simulink model "TST_CoEng_StEng"  (R2016b)
settings: Solver=FixedStepDiscrete  StartTime=0.0  StopTime=simTime  FixedStep=sampleTime  RelTol=1e-3
values from neighbouring files (symbols this model uses):
  testCase = 1    [initTST_CoEng_StEng_001.m]    (also in initTST_CoEng_StEng_002.m = 2; initTST_CoEng_StEng_003.m = 3; initTST_CoEng_StEng_004.m = 4; initTST_CoEng_StEng_005.m = 5)
libraries: simulink x41, UnitTest_Lib x25
(part 1 of 2)
settings Model: Creator=zhengjinyan  LastModifiedBy=zhengjinyan
settings DebuggingCC: SignalRangeChecking=error

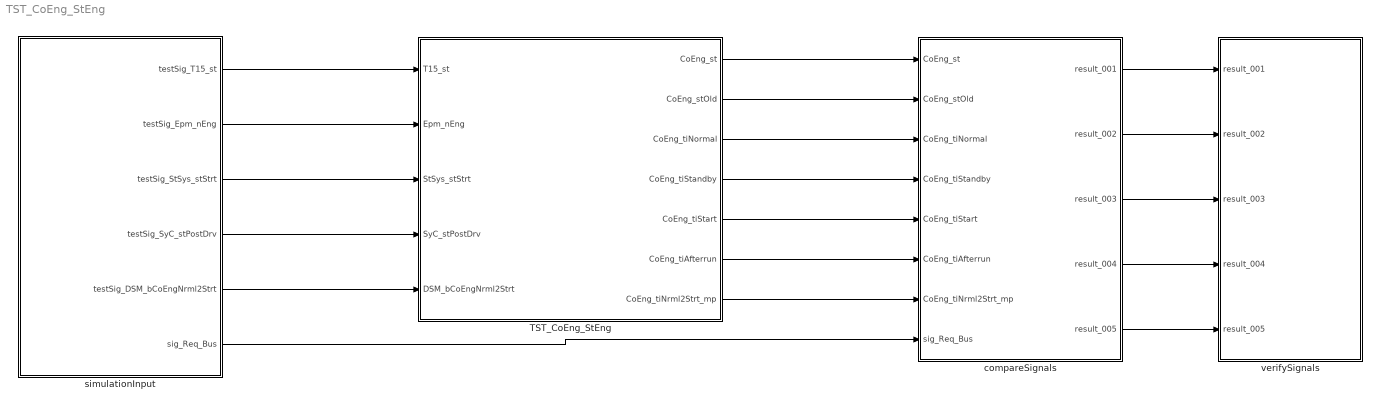
== system TST_CoEng_StEng ==
  TST_CoEng_StEng : Subsystem
  compareSignals : Subsystem
  simulationInput : Subsystem
  verifySignals : Subsystem
  wires:
  simulationInput/1(testSig_T15_st) -> TST_CoEng_StEng/1(T15_st)
  simulationInput/2(testSig_Epm_nEng) -> TST_CoEng_StEng/2(Epm_nEng)
  simulationInput/3(testSig_StSys_stStrt) -> TST_CoEng_StEng/3(StSys_stStrt)
  simulationInput/4(testSig_SyC_stPostDrv) -> TST_CoEng_StEng/4(SyC_stPostDrv)
  simulationInput/5(testSig_DSM_bCoEngNrml2Strt) -> TST_CoEng_StEng/5(DSM_bCoEngNrml2Strt)
  TST_CoEng_StEng/1(CoEng_st) -> compareSignals/1(CoEng_st)
  TST_CoEng_StEng/2(CoEng_stOld) -> compareSignals/2(CoEng_stOld)
  TST_CoEng_StEng/3(CoEng_tiNormal) -> compareSignals/3(CoEng_tiNormal)
  TST_CoEng_StEng/4(CoEng_tiStandby) -> compareSignals/4(CoEng_tiStandby)
  TST_CoEng_StEng/5(CoEng_tiStart) -> compareSignals/5(CoEng_tiStart)
  TST_CoEng_StEng/6(CoEng_tiAfterrun) -> compareSignals/6(CoEng_tiAfterrun)
  TST_CoEng_StEng/7(CoEng_tiNrml2Strt_mp) -> compareSignals/7(CoEng_tiNrml2Strt_mp)
  simulationInput/6(sig_Req_Bus) -> compareSignals/8(sig_Req_Bus)
  compareSignals/1(result_001) -> verifySignals/1(result_001)
  compareSignals/2(result_002) -> verifySignals/2(result_002)
  compareSignals/3(result_003) -> verifySignals/3(result_003)
  compareSignals/4(result_004) -> verifySignals/4(result_004)
  compareSignals/5(result_005) -> verifySignals/5(result_005)

== system TST_CoEng_StEng/TST_CoEng_StEng ==
  T15_st : Inport
  Epm_nEng : Inport  Port=2
  StSys_stStrt : Inport  Port=3
  SyC_stPostDrv : Inport  Port=4
  DSM_bCoEngNrml2Strt : Inport  Port=5
  CoEng_StEng : ModelReference  ModelNameDialog=CoEng_StEng  SimulationMode=Normal  ModelReferenceVersion=1.61  TriggerPortName=function  TriggerPortTriggerType=function-call  TriggerPortStatesWhenEnabling=held
  Function_Call : simulink/Ports & Subsystems/Function-Call Generator  sample_time=sampleTime  numberOfIterations=1
  CoEng_st : Outport
  CoEng_stOld : Outport  Port=2
  CoEng_tiNormal : Outport  Port=3
  CoEng_tiStandby : Outport  Port=4
  CoEng_tiStart : Outport  Port=5
  CoEng_tiAfterrun : Outport  Port=6
  CoEng_tiNrml2Strt_mp : Outport  Port=7
  wires:
  Function_Call/1 -> CoEng_StEng/Trigger
  T15_st/1 -> CoEng_StEng/1
  Epm_nEng/1 -> CoEng_StEng/2
  StSys_stStrt/1 -> CoEng_StEng/3
  SyC_stPostDrv/1 -> CoEng_StEng/4
  DSM_bCoEngNrml2Strt/1 -> CoEng_StEng/5
  CoEng_StEng/1 -> CoEng_st/1
  CoEng_StEng/2 -> CoEng_stOld/1
  CoEng_StEng/3 -> CoEng_tiNormal/1
  CoEng_StEng/4 -> CoEng_tiStandby/1
  CoEng_StEng/5 -> CoEng_tiStart/1
  CoEng_StEng/6 -> CoEng_tiAfterrun/1
  CoEng_StEng/7 -> CoEng_tiNrml2Strt_mp/1

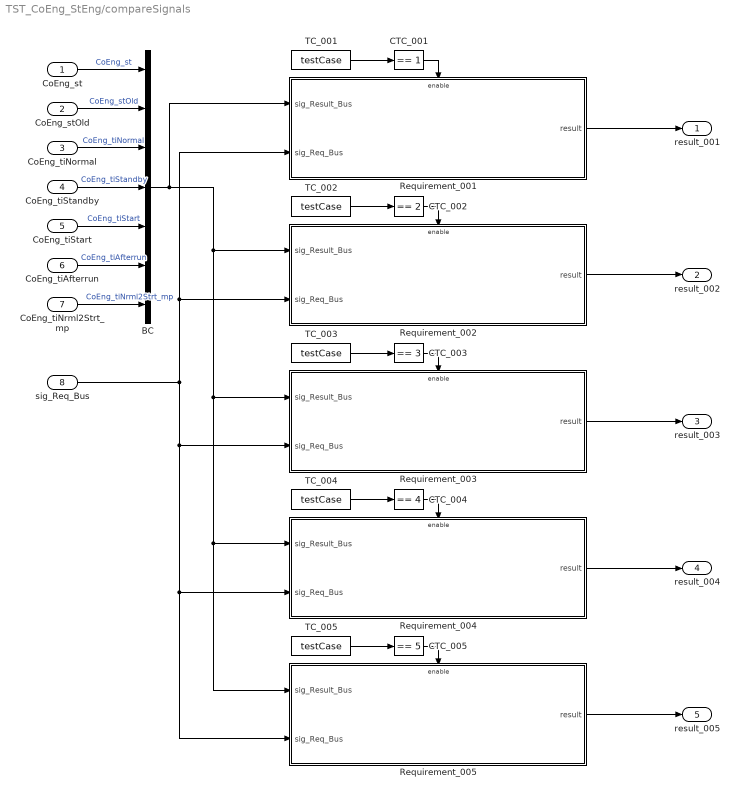
== system TST_CoEng_StEng/compareSignals ==
  CoEng_st : Inport
  CoEng_stOld : Inport  Port=2
  CoEng_tiNormal : Inport  Port=3
  CoEng_tiStandby : Inport  Port=4
  CoEng_tiStart : Inport  Port=5
  CoEng_tiAfterrun : Inport  Port=6
  CoEng_tiNrml2Strt_mp : Inport  Port=7
  sig_Req_Bus : Inport  Port=8
  BC : BusCreator  Inputs=7
  CTC_001 : simulink/Logic and Bit Operations/Compare To Constant  relop===  const=1  OutDataTypeStr=boolean
  CTC_002 : simulink/Logic and Bit Operations/Compare To Constant  relop===  const=2  OutDataTypeStr=boolean
  CTC_003 : simulink/Logic and Bit Operations/Compare To Constant  relop===  const=3  OutDataTypeStr=boolean
  CTC_004 : simulink/Logic and Bit Operations/Compare To Constant  relop===  const=4  OutDataTypeStr=boolean
  CTC_005 : simulink/Logic and Bit Operations/Compare To Constant  relop===  const=5  OutDataTypeStr=boolean
  Requirement_001 : Subsystem
  Requirement_002 : Subsystem
  Requirement_003 : Subsystem
  Requirement_004 : Subsystem
  Requirement_005 : Subsystem
  TC_001 : Constant  Value=testCase
  TC_002 : Constant  Value=testCase
  TC_003 : Constant  Value=testCase
  TC_004 : Constant  Value=testCase
  TC_005 : Constant  Value=testCase
  result_001 : Outport
  result_002 : Outport  Port=2
  result_003 : Outport  Port=3
  result_004 : Outport  Port=4
  result_005 : Outport  Port=5
  wires:
  CoEng_st/1 -> BC/1  "CoEng_st"
  CoEng_stOld/1 -> BC/2  "CoEng_stOld"
  CoEng_tiNormal/1 -> BC/3  "CoEng_tiNormal"
  CoEng_tiStandby/1 -> BC/4  "CoEng_tiStandby"
  CoEng_tiStart/1 -> BC/5  "CoEng_tiStart"
  CoEng_tiAfterrun/1 -> BC/6  "CoEng_tiAfterrun"
  CoEng_tiNrml2Strt_mp/1 -> BC/7  "CoEng_tiNrml2Strt_mp"
  TC_001/1 -> CTC_001/1
  CTC_001/1 -> Requirement_001/Enable
  sig_Req_Bus/1 -> Requirement_004/2(sig_Req_Bus), Requirement_005/2(sig_Req_Bus), Requirement_003/2(sig_Req_Bus), Requirement_001/2(sig_Req_Bus), Requirement_002/2(sig_Req_Bus)
  BC/1 -> Requirement_004/1(sig_Result_Bus), Requirement_005/1(sig_Result_Bus), Requirement_003/1(sig_Result_Bus), Requirement_002/1(sig_Result_Bus), Requirement_001/1(sig_Result_Bus)
  Requirement_001/1(result) -> result_001/1
  TC_002/1 -> CTC_002/1
  CTC_002/1 -> Requirement_002/Enable
  Requirement_002/1(result) -> result_002/1
  TC_003/1 -> CTC_003/1
  CTC_003/1 -> Requirement_003/Enable
  Requirement_003/1(result) -> result_003/1
  TC_004/1 -> CTC_004/1
  CTC_004/1 -> Requirement_004/Enable
  Requirement_004/1(result) -> result_004/1
  TC_005/1 -> CTC_005/1
  CTC_005/1 -> Requirement_005/Enable
  Requirement_005/1(result) -> result_005/1

== system TST_CoEng_StEng/simulationInput ==
  BS : BusSelector  OutputSignals=testSig_T15_st,testSig_Epm_nEng,testSig_StSys_stStrt,testSig_SyC_stPostDrv,testSig_DSM_bCoEngNrml2Strt
  MPSw : MultiPortSwitch  Inputs=5  SaturateOnIntegerOverflow=on  InputSameDT=on
  TestCase : Constant  Value=testCase
  testSignals_R001 : Subsystem
  testSignals_R002 : Subsystem
  testSignals_R003 : Subsystem
  testSignals_R004 : Subsystem
  testSignals_R005 : Subsystem
  testSig_T15_st : Outport
  testSig_Epm_nEng : Outport  Port=2
  testSig_StSys_stStrt : Outport  Port=3
  testSig_SyC_stPostDrv : Outport  Port=4
  testSig_DSM_bCoEngNrml2Strt : Outport  Port=5
  sig_Req_Bus : Outport  Port=6
  wires:
  BS/1 -> testSig_T15_st/1  "<testSig_T15_st>"
  BS/2 -> testSig_Epm_nEng/1  "<testSig_Epm_nEng>"
  BS/3 -> testSig_StSys_stStrt/1  "<testSig_StSys_stStrt>"
  BS/4 -> testSig_SyC_stPostDrv/1  "<testSig_SyC_stPostDrv>"
  BS/5 -> testSig_DSM_bCoEngNrml2Strt/1  "<testSig_DSM_bCoEngNrml2Strt>"
  MPSw/1 -> BS/1, sig_Req_Bus/1
  TestCase/1 -> MPSw/1
  testSignals_R001/1(testSignals) -> MPSw/2
  testSignals_R002/1(testSignals) -> MPSw/3
  testSignals_R003/1(testSignals) -> MPSw/4
  testSignals_R004/1(testSignals) -> MPSw/5
  testSignals_R005/1(testSignals) -> MPSw/6

== system TST_CoEng_StEng/verifySignals ==
  result_001 : Inport
  result_002 : Inport  Port=2
  result_003 : Inport  Port=3
  result_004 : Inport  Port=4
  result_005 : Inport  Port=5
  Assertion_001 : Assertion  Enabled=off
  Assertion_002 : Assertion  Enabled=off
  Assertion_003 : Assertion  Enabled=off
  Assertion_004 : Assertion  Enabled=off
  Assertion_005 : Assertion  Enabled=off
  wires:
  result_001/1 -> Assertion_001/1
  result_002/1 -> Assertion_002/1
  result_003/1 -> Assertion_003/1
  result_004/1 -> Assertion_004/1
  result_005/1 -> Assertion_005/1

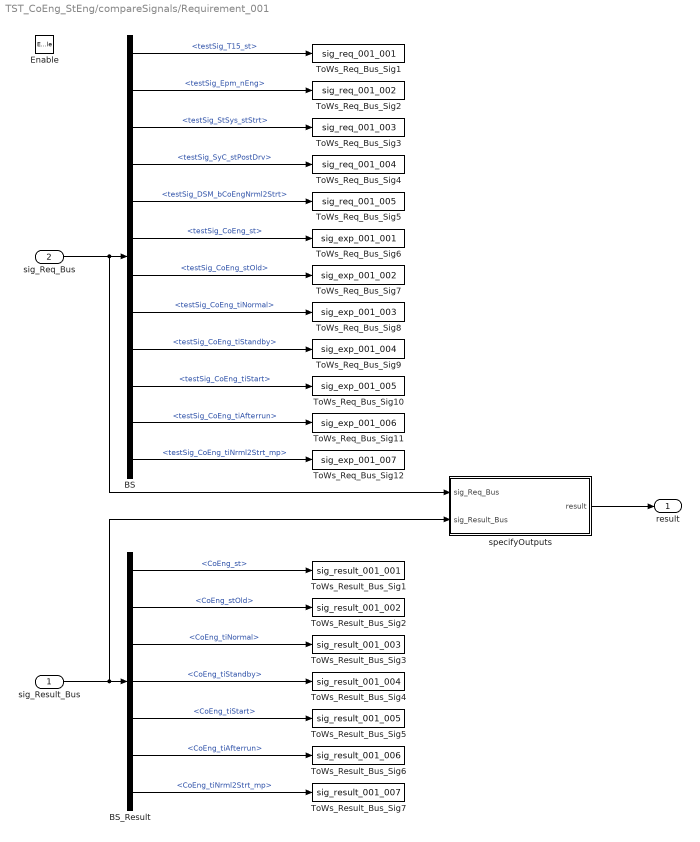
== system TST_CoEng_StEng/compareSignals/Requirement_001 ==
  sig_Result_Bus : Inport
  sig_Req_Bus : Inport  Port=2
  Enable : EnablePort
  BS : BusSelector  OutputSignals=testSig_T15_st,testSig_Epm_nEng,testSig_StSys_stStrt,testSig_SyC_stPostDrv,testSig_DSM_bCoEngNrml2Strt,testSig_CoEng_st,testSig_CoEng_stOld,testSig_CoEng_tiNormal,testSig_CoEng_tiStandby,testSig_CoEng_tiStart,testSig_CoEng_tiAfterrun,testSig_CoEng_tiNrml2Strt_mp
  BS_Result : BusSelector  OutputSignals=CoEng_st,CoEng_stOld,CoEng_tiNormal,CoEng_tiStandby,CoEng_tiStart,CoEng_tiAfterrun,CoEng_tiNrml2Strt_mp
  ToWs_Req_Bus_Sig1 : ToWorkspace  VariableName=sig_req_001_001  SaveFormat=Structure With Time
  ToWs_Req_Bus_Sig10 : ToWorkspace  VariableName=sig_exp_001_005  SaveFormat=Structure With Time
  ToWs_Req_Bus_Sig11 : ToWorkspace  VariableName=sig_exp_001_006  SaveFormat=Structure With Time
  ToWs_Req_Bus_Sig12 : ToWorkspace  VariableName=sig_exp_001_007  SaveFormat=Structure With Time
  ToWs_Req_Bus_Sig2 : ToWorkspace  VariableName=sig_req_001_002  SaveFormat=Structure With Time
  ToWs_Req_Bus_Sig3 : ToWorkspace  VariableName=sig_req_001_003  SaveFormat=Structure With Time
  ToWs_Req_Bus_Sig4 : ToWorkspace  VariableName=sig_req_001_004  SaveFormat=Structure With Time
  ToWs_Req_Bus_Sig5 : ToWorkspace  VariableName=sig_req_001_005  SaveFormat=Structure With Time
  ToWs_Req_Bus_Sig6 : ToWorkspace  VariableName=sig_exp_001_001  SaveFormat=Structure With Time
  ToWs_Req_Bus_Sig7 : ToWorkspace  VariableName=sig_exp_001_002  SaveFormat=Structure With Time
  ToWs_Req_Bus_Sig8 : ToWorkspace  VariableName=sig_exp_001_003  SaveFormat=Structure With Time
  ToWs_Req_Bus_Sig9 : ToWorkspace  VariableName=sig_exp_001_004  SaveFormat=Structure With Time
  ToWs_Result_Bus_Sig1 : ToWorkspace  VariableName=sig_result_001_001  SaveFormat=Structure With Time
  ToWs_Result_Bus_Sig2 : ToWorkspace  VariableName=sig_result_001_002  SaveFormat=Structure With Time
  ToWs_Result_Bus_Sig3 : ToWorkspace  VariableName=sig_result_001_003  SaveFormat=Structure With Time
  ToWs_Result_Bus_Sig4 : ToWorkspace  VariableName=sig_result_001_004  SaveFormat=Structure With Time
  ToWs_Result_Bus_Sig5 : ToWorkspace  VariableName=sig_result_001_005  SaveFormat=Structure With Time
  ToWs_Result_Bus_Sig6 : ToWorkspace  VariableName=sig_result_001_006  SaveFormat=Structure With Time
  ToWs_Result_Bus_Sig7 : ToWorkspace  VariableName=sig_result_001_007  SaveFormat=Structure With Time
  specifyOutputs : Subsystem
  result : Outport
  wires:
  sig_Req_Bus/1 -> BS/1, specifyOutputs/1(sig_Req_Bus)
  BS/1 -> ToWs_Req_Bus_Sig1/1  "<testSig_T15_st>"
  BS/2 -> ToWs_Req_Bus_Sig2/1  "<testSig_Epm_nEng>"
  BS/3 -> ToWs_Req_Bus_Sig3/1  "<testSig_StSys_stStrt>"
  BS/4 -> ToWs_Req_Bus_Sig4/1  "<testSig_SyC_stPostDrv>"
  BS/5 -> ToWs_Req_Bus_Sig5/1  "<testSig_DSM_bCoEngNrml2Strt>"
  BS/6 -> ToWs_Req_Bus_Sig6/1  "<testSig_CoEng_st>"
  BS/7 -> ToWs_Req_Bus_Sig7/1  "<testSig_CoEng_stOld>"
  BS/8 -> ToWs_Req_Bus_Sig8/1  "<testSig_CoEng_tiNormal>"
  BS/9 -> ToWs_Req_Bus_Sig9/1  "<testSig_CoEng_tiStandby>"
  BS/10 -> ToWs_Req_Bus_Sig10/1  "<testSig_CoEng_tiStart>"
  BS/11 -> ToWs_Req_Bus_Sig11/1  "<testSig_CoEng_tiAfterrun>"
  BS/12 -> ToWs_Req_Bus_Sig12/1  "<testSig_CoEng_tiNrml2Strt_mp>"
  sig_Result_Bus/1 -> BS_Result/1, specifyOutputs/2(sig_Result_Bus)
  BS_Result/1 -> ToWs_Result_Bus_Sig1/1  "<CoEng_st>"
  BS_Result/2 -> ToWs_Result_Bus_Sig2/1  "<CoEng_stOld>"
  BS_Result/3 -> ToWs_Result_Bus_Sig3/1  "<CoEng_tiNormal>"
  BS_Result/4 -> ToWs_Result_Bus_Sig4/1  "<CoEng_tiStandby>"
  BS_Result/5 -> ToWs_Result_Bus_Sig5/1  "<CoEng_tiStart>"
  BS_Result/6 -> ToWs_Result_Bus_Sig6/1  "<CoEng_tiAfterrun>"
  BS_Result/7 -> ToWs_Result_Bus_Sig7/1  "<CoEng_tiNrml2Strt_mp>"
  specifyOutputs/1(result) -> result/1

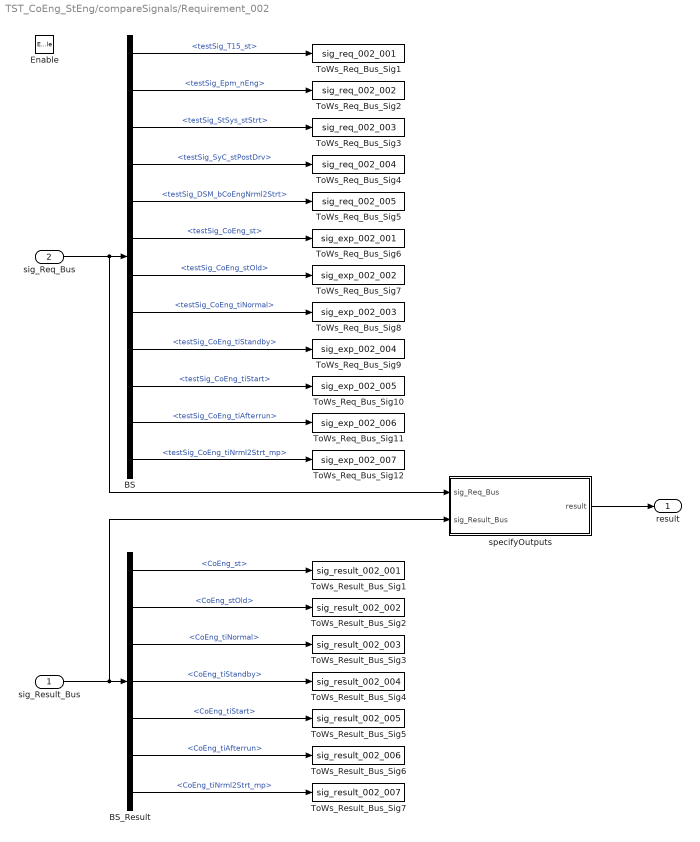
== system TST_CoEng_StEng/compareSignals/Requirement_002 ==
  sig_Result_Bus : Inport
  sig_Req_Bus : Inport  Port=2
  Enable : EnablePort
  BS : BusSelector  OutputSignals=testSig_T15_st,testSig_Epm_nEng,testSig_StSys_stStrt,testSig_SyC_stPostDrv,testSig_DSM_bCoEngNrml2Strt,testSig_CoEng_st,testSig_CoEng_stOld,testSig_CoEng_tiNormal,testSig_CoEng_tiStandby,testSig_CoEng_tiStart,testSig_CoEng_tiAfterrun,testSig_CoEng_tiNrml2Strt_mp
  BS_Result : BusSelector  OutputSignals=CoEng_st,CoEng_stOld,CoEng_tiNormal,CoEng_tiStandby,CoEng_tiStart,CoEng_tiAfterrun,CoEng_tiNrml2Strt_mp
  ToWs_Req_Bus_Sig1 : ToWorkspace  VariableName=sig_req_002_001  SaveFormat=Structure With Time
  ToWs_Req_Bus_Sig10 : ToWorkspace  VariableName=sig_exp_002_005  SaveFormat=Structure With Time
  ToWs_Req_Bus_Sig11 : ToWorkspace  VariableName=sig_exp_002_006  SaveFormat=Structure With Time
  ToWs_Req_Bus_Sig12 : ToWorkspace  VariableName=sig_exp_002_007  SaveFormat=Structure With Time
  ToWs_Req_Bus_Sig2 : ToWorkspace  VariableName=sig_req_002_002  SaveFormat=Structure With Time
  ToWs_Req_Bus_Sig3 : ToWorkspace  VariableName=sig_req_002_003  SaveFormat=Structure With Time
  ToWs_Req_Bus_Sig4 : ToWorkspace  VariableName=sig_req_002_004  SaveFormat=Structure With Time
  ToWs_Req_Bus_Sig5 : ToWorkspace  VariableName=sig_req_002_005  SaveFormat=Structure With Time
  ToWs_Req_Bus_Sig6 : ToWorkspace  VariableName=sig_exp_002_001  SaveFormat=Structure With Time
  ToWs_Req_Bus_Sig7 : ToWorkspace  VariableName=sig_exp_002_002  SaveFormat=Structure With Time
  ToWs_Req_Bus_Sig8 : ToWorkspace  VariableName=sig_exp_002_003  SaveFormat=Structure With Time
  ToWs_Req_Bus_Sig9 : ToWorkspace  VariableName=sig_exp_002_004  SaveFormat=Structure With Time
  ToWs_Result_Bus_Sig1 : ToWorkspace  VariableName=sig_result_002_001  SaveFormat=Structure With Time
  ToWs_Result_Bus_Sig2 : ToWorkspace  VariableName=sig_result_002_002  SaveFormat=Structure With Time
  ToWs_Result_Bus_Sig3 : ToWorkspace  VariableName=sig_result_002_003  SaveFormat=Structure With Time
  ToWs_Result_Bus_Sig4 : ToWorkspace  VariableName=sig_result_002_004  SaveFormat=Structure With Time
  ToWs_Result_Bus_Sig5 : ToWorkspace  VariableName=sig_result_002_005  SaveFormat=Structure With Time
  ToWs_Result_Bus_Sig6 : ToWorkspace  VariableName=sig_result_002_006  SaveFormat=Structure With Time
  ToWs_Result_Bus_Sig7 : ToWorkspace  VariableName=sig_result_002_007  SaveFormat=Structure With Time
  specifyOutputs : Subsystem
  result : Outport
  wires:
  sig_Req_Bus/1 -> BS/1, specifyOutputs/1(sig_Req_Bus)
  BS/1 -> ToWs_Req_Bus_Sig1/1  "<testSig_T15_st>"
  BS/2 -> ToWs_Req_Bus_Sig2/1  "<testSig_Epm_nEng>"
  BS/3 -> ToWs_Req_Bus_Sig3/1  "<testSig_StSys_stStrt>"
  BS/4 -> ToWs_Req_Bus_Sig4/1  "<testSig_SyC_stPostDrv>"
  BS/5 -> ToWs_Req_Bus_Sig5/1  "<testSig_DSM_bCoEngNrml2Strt>"
  BS/6 -> ToWs_Req_Bus_Sig6/1  "<testSig_CoEng_st>"
  BS/7 -> ToWs_Req_Bus_Sig7/1  "<testSig_CoEng_stOld>"
  BS/8 -> ToWs_Req_Bus_Sig8/1  "<testSig_CoEng_tiNormal>"
  BS/9 -> ToWs_Req_Bus_Sig9/1  "<testSig_CoEng_tiStandby>"
  BS/10 -> ToWs_Req_Bus_Sig10/1  "<testSig_CoEng_tiStart>"
  BS/11 -> ToWs_Req_Bus_Sig11/1  "<testSig_CoEng_tiAfterrun>"
  BS/12 -> ToWs_Req_Bus_Sig12/1  "<testSig_CoEng_tiNrml2Strt_mp>"
  sig_Result_Bus/1 -> BS_Result/1, specifyOutputs/2(sig_Result_Bus)
  BS_Result/1 -> ToWs_Result_Bus_Sig1/1  "<CoEng_st>"
  BS_Result/2 -> ToWs_Result_Bus_Sig2/1  "<CoEng_stOld>"
  BS_Result/3 -> ToWs_Result_Bus_Sig3/1  "<CoEng_tiNormal>"
  BS_Result/4 -> ToWs_Result_Bus_Sig4/1  "<CoEng_tiStandby>"
  BS_Result/5 -> ToWs_Result_Bus_Sig5/1  "<CoEng_tiStart>"
  BS_Result/6 -> ToWs_Result_Bus_Sig6/1  "<CoEng_tiAfterrun>"
  BS_Result/7 -> ToWs_Result_Bus_Sig7/1  "<CoEng_tiNrml2Strt_mp>"
  specifyOutputs/1(result) -> result/1

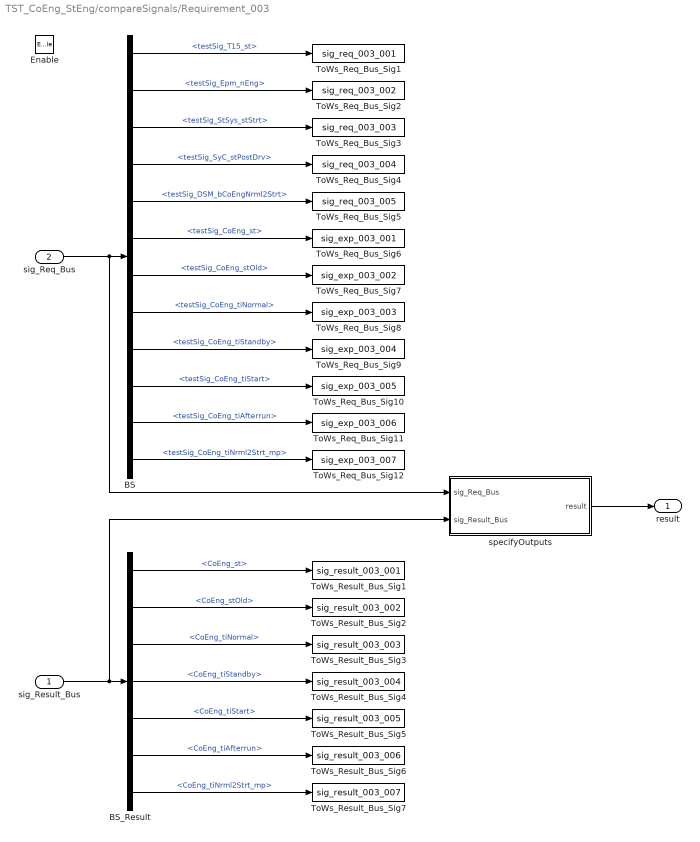
== system TST_CoEng_StEng/compareSignals/Requirement_003 ==
  sig_Result_Bus : Inport
  sig_Req_Bus : Inport  Port=2
  Enable : EnablePort
  BS : BusSelector  OutputSignals=testSig_T15_st,testSig_Epm_nEng,testSig_StSys_stStrt,testSig_SyC_stPostDrv,testSig_DSM_bCoEngNrml2Strt,testSig_CoEng_st,testSig_CoEng_stOld,testSig_CoEng_tiNormal,testSig_CoEng_tiStandby,testSig_CoEng_tiStart,testSig_CoEng_tiAfterrun,testSig_CoEng_tiNrml2Strt_mp
  BS_Result : BusSelector  OutputSignals=CoEng_st,CoEng_stOld,CoEng_tiNormal,CoEng_tiStandby,CoEng_tiStart,CoEng_tiAfterrun,CoEng_tiNrml2Strt_mp
  ToWs_Req_Bus_Sig1 : ToWorkspace  VariableName=sig_req_003_001  SaveFormat=Structure With Time
  ToWs_Req_Bus_Sig10 : ToWorkspace  VariableName=sig_exp_003_005  SaveFormat=Structure With Time
  ToWs_Req_Bus_Sig11 : ToWorkspace  VariableName=sig_exp_003_006  SaveFormat=Structure With Time
  ToWs_Req_Bus_Sig12 : ToWorkspace  VariableName=sig_exp_003_007  SaveFormat=Structure With Time
  ToWs_Req_Bus_Sig2 : ToWorkspace  VariableName=sig_req_003_002  SaveFormat=Structure With Time
  ToWs_Req_Bus_Sig3 : ToWorkspace  VariableName=sig_req_003_003  SaveFormat=Structure With Time
  ToWs_Req_Bus_Sig4 : ToWorkspace  VariableName=sig_req_003_004  SaveFormat=Structure With Time
  ToWs_Req_Bus_Sig5 : ToWorkspace  VariableName=sig_req_003_005  SaveFormat=Structure With Time
  ToWs_Req_Bus_Sig6 : ToWorkspace  VariableName=sig_exp_003_001  SaveFormat=Structure With Time
  ToWs_Req_Bus_Sig7 : ToWorkspace  VariableName=sig_exp_003_002  SaveFormat=Structure With Time
  ToWs_Req_Bus_Sig8 : ToWorkspace  VariableName=sig_exp_003_003  SaveFormat=Structure With Time
  ToWs_Req_Bus_Sig9 : ToWorkspace  VariableName=sig_exp_003_004  SaveFormat=Structure With Time
  ToWs_Result_Bus_Sig1 : ToWorkspace  VariableName=sig_result_003_001  SaveFormat=Structure With Time
  ToWs_Result_Bus_Sig2 : ToWorkspace  VariableName=sig_result_003_002  SaveFormat=Structure With Time
  ToWs_Result_Bus_Sig3 : ToWorkspace  VariableName=sig_result_003_003  SaveFormat=Structure With Time
  ToWs_Result_Bus_Sig4 : ToWorkspace  VariableName=sig_result_003_004  SaveFormat=Structure With Time
  ToWs_Result_Bus_Sig5 : ToWorkspace  VariableName=sig_result_003_005  SaveFormat=Structure With Time
  ToWs_Result_Bus_Sig6 : ToWorkspace  VariableName=sig_result_003_006  SaveFormat=Structure With Time
  ToWs_Result_Bus_Sig7 : ToWorkspace  VariableName=sig_result_003_007  SaveFormat=Structure With Time
  specifyOutputs : Subsystem
  result : Outport
  wires:
  sig_Req_Bus/1 -> BS/1, specifyOutputs/1(sig_Req_Bus)
  BS/1 -> ToWs_Req_Bus_Sig1/1  "<testSig_T15_st>"
  BS/2 -> ToWs_Req_Bus_Sig2/1  "<testSig_Epm_nEng>"
  BS/3 -> ToWs_Req_Bus_Sig3/1  "<testSig_StSys_stStrt>"
  BS/4 -> ToWs_Req_Bus_Sig4/1  "<testSig_SyC_stPostDrv>"
  BS/5 -> ToWs_Req_Bus_Sig5/1  "<testSig_DSM_bCoEngNrml2Strt>"
  BS/6 -> ToWs_Req_Bus_Sig6/1  "<testSig_CoEng_st>"
  BS/7 -> ToWs_Req_Bus_Sig7/1  "<testSig_CoEng_stOld>"
  BS/8 -> ToWs_Req_Bus_Sig8/1  "<testSig_CoEng_tiNormal>"
  BS/9 -> ToWs_Req_Bus_Sig9/1  "<testSig_CoEng_tiStandby>"
  BS/10 -> ToWs_Req_Bus_Sig10/1  "<testSig_CoEng_tiStart>"
  BS/11 -> ToWs_Req_Bus_Sig11/1  "<testSig_CoEng_tiAfterrun>"
  BS/12 -> ToWs_Req_Bus_Sig12/1  "<testSig_CoEng_tiNrml2Strt_mp>"
  sig_Result_Bus/1 -> BS_Result/1, specifyOutputs/2(sig_Result_Bus)
  BS_Result/1 -> ToWs_Result_Bus_Sig1/1  "<CoEng_st>"
  BS_Result/2 -> ToWs_Result_Bus_Sig2/1  "<CoEng_stOld>"
  BS_Result/3 -> ToWs_Result_Bus_Sig3/1  "<CoEng_tiNormal>"
  BS_Result/4 -> ToWs_Result_Bus_Sig4/1  "<CoEng_tiStandby>"
  BS_Result/5 -> ToWs_Result_Bus_Sig5/1  "<CoEng_tiStart>"
  BS_Result/6 -> ToWs_Result_Bus_Sig6/1  "<CoEng_tiAfterrun>"
  BS_Result/7 -> ToWs_Result_Bus_Sig7/1  "<CoEng_tiNrml2Strt_mp>"
  specifyOutputs/1(result) -> result/1

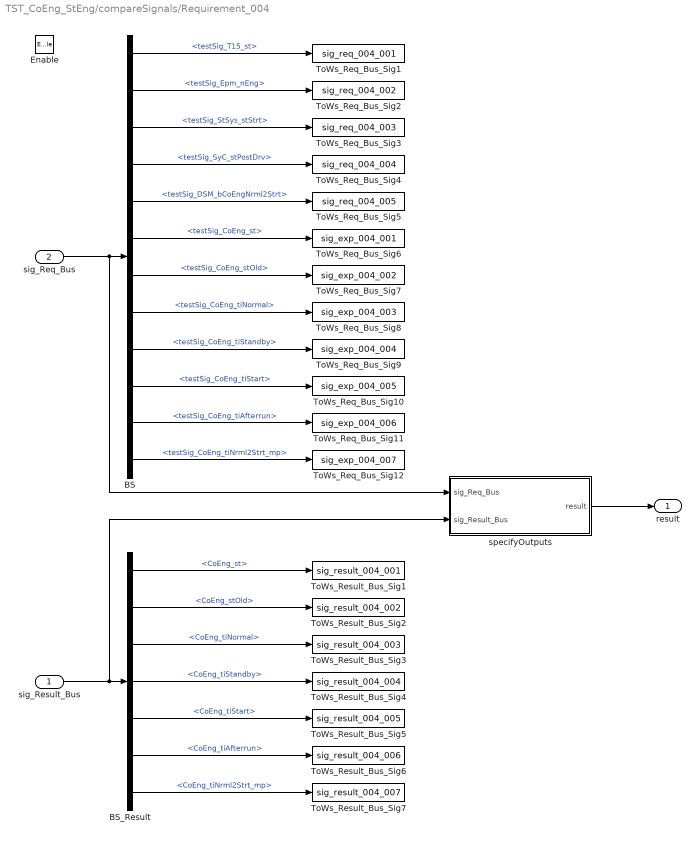
== system TST_CoEng_StEng/compareSignals/Requirement_004 ==
  sig_Result_Bus : Inport
  sig_Req_Bus : Inport  Port=2
  Enable : EnablePort
  BS : BusSelector  OutputSignals=testSig_T15_st,testSig_Epm_nEng,testSig_StSys_stStrt,testSig_SyC_stPostDrv,testSig_DSM_bCoEngNrml2Strt,testSig_CoEng_st,testSig_CoEng_stOld,testSig_CoEng_tiNormal,testSig_CoEng_tiStandby,testSig_CoEng_tiStart,testSig_CoEng_tiAfterrun,testSig_CoEng_tiNrml2Strt_mp
  BS_Result : BusSelector  OutputSignals=CoEng_st,CoEng_stOld,CoEng_tiNormal,CoEng_tiStandby,CoEng_tiStart,CoEng_tiAfterrun,CoEng_tiNrml2Strt_mp
  ToWs_Req_Bus_Sig1 : ToWorkspace  VariableName=sig_req_004_001  SaveFormat=Structure With Time
  ToWs_Req_Bus_Sig10 : ToWorkspace  VariableName=sig_exp_004_005  SaveFormat=Structure With Time
  ToWs_Req_Bus_Sig11 : ToWorkspace  VariableName=sig_exp_004_006  SaveFormat=Structure With Time
  ToWs_Req_Bus_Sig12 : ToWorkspace  VariableName=sig_exp_004_007  SaveFormat=Structure With Time
  ToWs_Req_Bus_Sig2 : ToWorkspace  VariableName=sig_req_004_002  SaveFormat=Structure With Time
  ToWs_Req_Bus_Sig3 : ToWorkspace  VariableName=sig_req_004_003  SaveFormat=Structure With Time
  ToWs_Req_Bus_Sig4 : ToWorkspace  VariableName=sig_req_004_004  SaveFormat=Structure With Time
  ToWs_Req_Bus_Sig5 : ToWorkspace  VariableName=sig_req_004_005  SaveFormat=Structure With Time
  ToWs_Req_Bus_Sig6 : ToWorkspace  VariableName=sig_exp_004_001  SaveFormat=Structure With Time
  ToWs_Req_Bus_Sig7 : ToWorkspace  VariableName=sig_exp_004_002  SaveFormat=Structure With Time
  ToWs_Req_Bus_Sig8 : ToWorkspace  VariableName=sig_exp_004_003  SaveFormat=Structure With Time
  ToWs_Req_Bus_Sig9 : ToWorkspace  VariableName=sig_exp_004_004  SaveFormat=Structure With Time
  ToWs_Result_Bus_Sig1 : ToWorkspace  VariableName=sig_result_004_001  SaveFormat=Structure With Time
  ToWs_Result_Bus_Sig2 : ToWorkspace  VariableName=sig_result_004_002  SaveFormat=Structure With Time
  ToWs_Result_Bus_Sig3 : ToWorkspace  VariableName=sig_result_004_003  SaveFormat=Structure With Time
  ToWs_Result_Bus_Sig4 : ToWorkspace  VariableName=sig_result_004_004  SaveFormat=Structure With Time
  ToWs_Result_Bus_Sig5 : ToWorkspace  VariableName=sig_result_004_005  SaveFormat=Structure With Time
  ToWs_Result_Bus_Sig6 : ToWorkspace  VariableName=sig_result_004_006  SaveFormat=Structure With Time
  ToWs_Result_Bus_Sig7 : ToWorkspace  VariableName=sig_result_004_007  SaveFormat=Structure With Time
  specifyOutputs : Subsystem
  result : Outport
  wires:
  sig_Req_Bus/1 -> BS/1, specifyOutputs/1(sig_Req_Bus)
  BS/1 -> ToWs_Req_Bus_Sig1/1  "<testSig_T15_st>"
  BS/2 -> ToWs_Req_Bus_Sig2/1  "<testSig_Epm_nEng>"
  BS/3 -> ToWs_Req_Bus_Sig3/1  "<testSig_StSys_stStrt>"
  BS/4 -> ToWs_Req_Bus_Sig4/1  "<testSig_SyC_stPostDrv>"
  BS/5 -> ToWs_Req_Bus_Sig5/1  "<testSig_DSM_bCoEngNrml2Strt>"
  BS/6 -> ToWs_Req_Bus_Sig6/1  "<testSig_CoEng_st>"
  BS/7 -> ToWs_Req_Bus_Sig7/1  "<testSig_CoEng_stOld>"
  BS/8 -> ToWs_Req_Bus_Sig8/1  "<testSig_CoEng_tiNormal>"
  BS/9 -> ToWs_Req_Bus_Sig9/1  "<testSig_CoEng_tiStandby>"
  BS/10 -> ToWs_Req_Bus_Sig10/1  "<testSig_CoEng_tiStart>"
  BS/11 -> ToWs_Req_Bus_Sig11/1  "<testSig_CoEng_tiAfterrun>"
  BS/12 -> ToWs_Req_Bus_Sig12/1  "<testSig_CoEng_tiNrml2Strt_mp>"
  sig_Result_Bus/1 -> BS_Result/1, specifyOutputs/2(sig_Result_Bus)
  BS_Result/1 -> ToWs_Result_Bus_Sig1/1  "<CoEng_st>"
  BS_Result/2 -> ToWs_Result_Bus_Sig2/1  "<CoEng_stOld>"
  BS_Result/3 -> ToWs_Result_Bus_Sig3/1  "<CoEng_tiNormal>"
  BS_Result/4 -> ToWs_Result_Bus_Sig4/1  "<CoEng_tiStandby>"
  BS_Result/5 -> ToWs_Result_Bus_Sig5/1  "<CoEng_tiStart>"
  BS_Result/6 -> ToWs_Result_Bus_Sig6/1  "<CoEng_tiAfterrun>"
  BS_Result/7 -> ToWs_Result_Bus_Sig7/1  "<CoEng_tiNrml2Strt_mp>"
  specifyOutputs/1(result) -> result/1

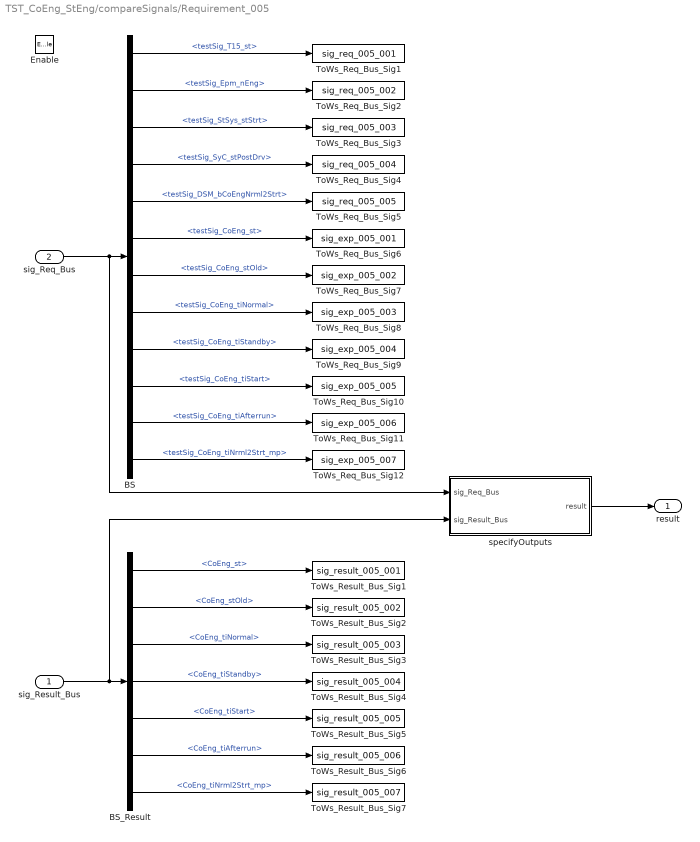
== system TST_CoEng_StEng/compareSignals/Requirement_005 ==
  sig_Result_Bus : Inport
  sig_Req_Bus : Inport  Port=2
  Enable : EnablePort
  BS : BusSelector  OutputSignals=testSig_T15_st,testSig_Epm_nEng,testSig_StSys_stStrt,testSig_SyC_stPostDrv,testSig_DSM_bCoEngNrml2Strt,testSig_CoEng_st,testSig_CoEng_stOld,testSig_CoEng_tiNormal,testSig_CoEng_tiStandby,testSig_CoEng_tiStart,testSig_CoEng_tiAfterrun,testSig_CoEng_tiNrml2Strt_mp
  BS_Result : BusSelector  OutputSignals=CoEng_st,CoEng_stOld,CoEng_tiNormal,CoEng_tiStandby,CoEng_tiStart,CoEng_tiAfterrun,CoEng_tiNrml2Strt_mp
  ToWs_Req_Bus_Sig1 : ToWorkspace  VariableName=sig_req_005_001  SaveFormat=Structure With Time
  ToWs_Req_Bus_Sig10 : ToWorkspace  VariableName=sig_exp_005_005  SaveFormat=Structure With Time
  ToWs_Req_Bus_Sig11 : ToWorkspace  VariableName=sig_exp_005_006  SaveFormat=Structure With Time
  ToWs_Req_Bus_Sig12 : ToWorkspace  VariableName=sig_exp_005_007  SaveFormat=Structure With Time
  ToWs_Req_Bus_Sig2 : ToWorkspace  VariableName=sig_req_005_002  SaveFormat=Structure With Time
  ToWs_Req_Bus_Sig3 : ToWorkspace  VariableName=sig_req_005_003  SaveFormat=Structure With Time
  ToWs_Req_Bus_Sig4 : ToWorkspace  VariableName=sig_req_005_004  SaveFormat=Structure With Time
  ToWs_Req_Bus_Sig5 : ToWorkspace  VariableName=sig_req_005_005  SaveFormat=Structure With Time
  ToWs_Req_Bus_Sig6 : ToWorkspace  VariableName=sig_exp_005_001  SaveFormat=Structure With Time
  ToWs_Req_Bus_Sig7 : ToWorkspace  VariableName=sig_exp_005_002  SaveFormat=Structure With Time
  ToWs_Req_Bus_Sig8 : ToWorkspace  VariableName=sig_exp_005_003  SaveFormat=Structure With Time
  ToWs_Req_Bus_Sig9 : ToWorkspace  VariableName=sig_exp_005_004  SaveFormat=Structure With Time
  ToWs_Result_Bus_Sig1 : ToWorkspace  VariableName=sig_result_005_001  SaveFormat=Structure With Time
  ToWs_Result_Bus_Sig2 : ToWorkspace  VariableName=sig_result_005_002  SaveFormat=Structure With Time
  ToWs_Result_Bus_Sig3 : ToWorkspace  VariableName=sig_result_005_003  SaveFormat=Structure With Time
  ToWs_Result_Bus_Sig4 : ToWorkspace  VariableName=sig_result_005_004  SaveFormat=Structure With Time
  ToWs_Result_Bus_Sig5 : ToWorkspace  VariableName=sig_result_005_005  SaveFormat=Structure With Time
  ToWs_Result_Bus_Sig6 : ToWorkspace  VariableName=sig_result_005_006  SaveFormat=Structure With Time
  ToWs_Result_Bus_Sig7 : ToWorkspace  VariableName=sig_result_005_007  SaveFormat=Structure With Time
  specifyOutputs : Subsystem
  result : Outport
  wires:
  sig_Req_Bus/1 -> BS/1, specifyOutputs/1(sig_Req_Bus)
  BS/1 -> ToWs_Req_Bus_Sig1/1  "<testSig_T15_st>"
  BS/2 -> ToWs_Req_Bus_Sig2/1  "<testSig_Epm_nEng>"
  BS/3 -> ToWs_Req_Bus_Sig3/1  "<testSig_StSys_stStrt>"
  BS/4 -> ToWs_Req_Bus_Sig4/1  "<testSig_SyC_stPostDrv>"
  BS/5 -> ToWs_Req_Bus_Sig5/1  "<testSig_DSM_bCoEngNrml2Strt>"
  BS/6 -> ToWs_Req_Bus_Sig6/1  "<testSig_CoEng_st>"
  BS/7 -> ToWs_Req_Bus_Sig7/1  "<testSig_CoEng_stOld>"
  BS/8 -> ToWs_Req_Bus_Sig8/1  "<testSig_CoEng_tiNormal>"
  BS/9 -> ToWs_Req_Bus_Sig9/1  "<testSig_CoEng_tiStandby>"
  BS/10 -> ToWs_Req_Bus_Sig10/1  "<testSig_CoEng_tiStart>"
  BS/11 -> ToWs_Req_Bus_Sig11/1  "<testSig_CoEng_tiAfterrun>"
  BS/12 -> ToWs_Req_Bus_Sig12/1  "<testSig_CoEng_tiNrml2Strt_mp>"
  sig_Result_Bus/1 -> BS_Result/1, specifyOutputs/2(sig_Result_Bus)
  BS_Result/1 -> ToWs_Result_Bus_Sig1/1  "<CoEng_st>"
  BS_Result/2 -> ToWs_Result_Bus_Sig2/1  "<CoEng_stOld>"
  BS_Result/3 -> ToWs_Result_Bus_Sig3/1  "<CoEng_tiNormal>"
  BS_Result/4 -> ToWs_Result_Bus_Sig4/1  "<CoEng_tiStandby>"
  BS_Result/5 -> ToWs_Result_Bus_Sig5/1  "<CoEng_tiStart>"
  BS_Result/6 -> ToWs_Result_Bus_Sig6/1  "<CoEng_tiAfterrun>"
  BS_Result/7 -> ToWs_Result_Bus_Sig7/1  "<CoEng_tiNrml2Strt_mp>"
  specifyOutputs/1(result) -> result/1

== system TST_CoEng_StEng/simulationInput/testSignals_R001 ==
  BC : BusCreator  Inputs=12
  spec_CoEng_st : FromWorkspace  VariableName=testSig_CoEng_st  Interpolate=off  OutputAfterFinalValue=Holding final value
  spec_CoEng_stOld : FromWorkspace  VariableName=testSig_CoEng_stOld  Interpolate=off  OutputAfterFinalValue=Holding final value
  spec_CoEng_tiAfterrun : FromWorkspace  VariableName=testSig_CoEng_tiAfterrun  Interpolate=off  OutputAfterFinalValue=Holding final value
  spec_CoEng_tiNormal : FromWorkspace  VariableName=testSig_CoEng_tiNormal  Interpolate=off  OutputAfterFinalValue=Holding final value
  spec_CoEng_tiNrml2Strt_mp : FromWorkspace  VariableName=testSig_CoEng_tiNrml2Strt_mp  Interpolate=off  OutputAfterFinalValue=Holding final value
  spec_CoEng_tiStandby : FromWorkspace  VariableName=testSig_CoEng_tiStandby  Interpolate=off  OutputAfterFinalValue=Holding final value
  spec_CoEng_tiStart : FromWorkspace  VariableName=testSig_CoEng_tiStart  Interpolate=off  OutputAfterFinalValue=Holding final value
  spec_DSM_bCoEngNrml2Strt : FromWorkspace  VariableName=testSig_DSM_bCoEngNrml2Strt  Interpolate=off  OutputAfterFinalValue=Holding final value
  spec_Epm_nEng : FromWorkspace  VariableName=testSig_Epm_nEng  Interpolate=off  OutputAfterFinalValue=Holding final value
  spec_StSys_stStrt : FromWorkspace  VariableName=testSig_StSys_stStrt  Interpolate=off  OutputAfterFinalValue=Holding final value
  spec_SyC_stPostDrv : FromWorkspace  VariableName=testSig_SyC_stPostDrv  Interpolate=off  OutputAfterFinalValue=Holding final value
  spec_T15_st : FromWorkspace  VariableName=testSig_T15_st  Interpolate=off  OutputAfterFinalValue=Holding final value
  testSignals : Outport
  wires:
  BC/1 -> testSignals/1
  spec_T15_st/1 -> BC/1  "testSig_T15_st"
  spec_Epm_nEng/1 -> BC/2  "testSig_Epm_nEng"
  spec_StSys_stStrt/1 -> BC/3  "testSig_StSys_stStrt"
  spec_SyC_stPostDrv/1 -> BC/4  "testSig_SyC_stPostDrv"
  spec_DSM_bCoEngNrml2Strt/1 -> BC/5  "testSig_DSM_bCoEngNrml2Strt"
  spec_CoEng_st/1 -> BC/6  "testSig_CoEng_st"
  spec_CoEng_stOld/1 -> BC/7  "testSig_CoEng_stOld"
  spec_CoEng_tiNormal/1 -> BC/8  "testSig_CoEng_tiNormal"
  spec_CoEng_tiStandby/1 -> BC/9  "testSig_CoEng_tiStandby"
  spec_CoEng_tiStart/1 -> BC/10  "testSig_CoEng_tiStart"
  spec_CoEng_tiAfterrun/1 -> BC/11  "testSig_CoEng_tiAfterrun"
  spec_CoEng_tiNrml2Strt_mp/1 -> BC/12  "testSig_CoEng_tiNrml2Strt_mp"

== system TST_CoEng_StEng/simulationInput/testSignals_R002 ==
  BC : BusCreator  Inputs=12
  spec_CoEng_st : FromWorkspace  VariableName=testSig_CoEng_st  Interpolate=off  OutputAfterFinalValue=Holding final value
  spec_CoEng_stOld : FromWorkspace  VariableName=testSig_CoEng_stOld  Interpolate=off  OutputAfterFinalValue=Holding final value
  spec_CoEng_tiAfterrun : FromWorkspace  VariableName=testSig_CoEng_tiAfterrun  Interpolate=off  OutputAfterFinalValue=Holding final value
  spec_CoEng_tiNormal : FromWorkspace  VariableName=testSig_CoEng_tiNormal  Interpolate=off  OutputAfterFinalValue=Holding final value
  spec_CoEng_tiNrml2Strt_mp : FromWorkspace  VariableName=testSig_CoEng_tiNrml2Strt_mp  Interpolate=off  OutputAfterFinalValue=Holding final value
  spec_CoEng_tiStandby : FromWorkspace  VariableName=testSig_CoEng_tiStandby  Interpolate=off  OutputAfterFinalValue=Holding final value
  spec_CoEng_tiStart : FromWorkspace  VariableName=testSig_CoEng_tiStart  Interpolate=off  OutputAfterFinalValue=Holding final value
  spec_DSM_bCoEngNrml2Strt : FromWorkspace  VariableName=testSig_DSM_bCoEngNrml2Strt  Interpolate=off  OutputAfterFinalValue=Holding final value
  spec_Epm_nEng : FromWorkspace  VariableName=testSig_Epm_nEng  Interpolate=off  OutputAfterFinalValue=Holding final value
  spec_StSys_stStrt : FromWorkspace  VariableName=testSig_StSys_stStrt  Interpolate=off  OutputAfterFinalValue=Holding final value
  spec_SyC_stPostDrv : FromWorkspace  VariableName=testSig_SyC_stPostDrv  Interpolate=off  OutputAfterFinalValue=Holding final value
  spec_T15_st : FromWorkspace  VariableName=testSig_T15_st  Interpolate=off  OutputAfterFinalValue=Holding final value
  testSignals : Outport
  wires:
  BC/1 -> testSignals/1
  spec_T15_st/1 -> BC/1  "testSig_T15_st"
  spec_Epm_nEng/1 -> BC/2  "testSig_Epm_nEng"
  spec_StSys_stStrt/1 -> BC/3  "testSig_StSys_stStrt"
  spec_SyC_stPostDrv/1 -> BC/4  "testSig_SyC_stPostDrv"
  spec_DSM_bCoEngNrml2Strt/1 -> BC/5  "testSig_DSM_bCoEngNrml2Strt"
  spec_CoEng_st/1 -> BC/6  "testSig_CoEng_st"
  spec_CoEng_stOld/1 -> BC/7  "testSig_CoEng_stOld"
  spec_CoEng_tiNormal/1 -> BC/8  "testSig_CoEng_tiNormal"
  spec_CoEng_tiStandby/1 -> BC/9  "testSig_CoEng_tiStandby"
  spec_CoEng_tiStart/1 -> BC/10  "testSig_CoEng_tiStart"
  spec_CoEng_tiAfterrun/1 -> BC/11  "testSig_CoEng_tiAfterrun"
  spec_CoEng_tiNrml2Strt_mp/1 -> BC/12  "testSig_CoEng_tiNrml2Strt_mp"

== system TST_CoEng_StEng/simulationInput/testSignals_R003 ==
  BC : BusCreator  Inputs=12
  spec_CoEng_st : FromWorkspace  VariableName=testSig_CoEng_st  Interpolate=off  OutputAfterFinalValue=Holding final value
  spec_CoEng_stOld : FromWorkspace  VariableName=testSig_CoEng_stOld  Interpolate=off  OutputAfterFinalValue=Holding final value
  spec_CoEng_tiAfterrun : FromWorkspace  VariableName=testSig_CoEng_tiAfterrun  Interpolate=off  OutputAfterFinalValue=Holding final value
  spec_CoEng_tiNormal : FromWorkspace  VariableName=testSig_CoEng_tiNormal  Interpolate=off  OutputAfterFinalValue=Holding final value
  spec_CoEng_tiNrml2Strt_mp : FromWorkspace  VariableName=testSig_CoEng_tiNrml2Strt_mp  Interpolate=off  OutputAfterFinalValue=Holding final value
  spec_CoEng_tiStandby : FromWorkspace  VariableName=testSig_CoEng_tiStandby  Interpolate=off  OutputAfterFinalValue=Holding final value
  spec_CoEng_tiStart : FromWorkspace  VariableName=testSig_CoEng_tiStart  Interpolate=off  OutputAfterFinalValue=Holding final value
  spec_DSM_bCoEngNrml2Strt : FromWorkspace  VariableName=testSig_DSM_bCoEngNrml2Strt  Interpolate=off  OutputAfterFinalValue=Holding final value
  spec_Epm_nEng : FromWorkspace  VariableName=testSig_Epm_nEng  Interpolate=off  OutputAfterFinalValue=Holding final value
  spec_StSys_stStrt : FromWorkspace  VariableName=testSig_StSys_stStrt  Interpolate=off  OutputAfterFinalValue=Holding final value
  spec_SyC_stPostDrv : FromWorkspace  VariableName=testSig_SyC_stPostDrv  Interpolate=off  OutputAfterFinalValue=Holding final value
  spec_T15_st : FromWorkspace  VariableName=testSig_T15_st  Interpolate=off  OutputAfterFinalValue=Holding final value
  testSignals : Outport
  wires:
  BC/1 -> testSignals/1
  spec_T15_st/1 -> BC/1  "testSig_T15_st"
  spec_Epm_nEng/1 -> BC/2  "testSig_Epm_nEng"
  spec_StSys_stStrt/1 -> BC/3  "testSig_StSys_stStrt"
  spec_SyC_stPostDrv/1 -> BC/4  "testSig_SyC_stPostDrv"
  spec_DSM_bCoEngNrml2Strt/1 -> BC/5  "testSig_DSM_bCoEngNrml2Strt"
  spec_CoEng_st/1 -> BC/6  "testSig_CoEng_st"
  spec_CoEng_stOld/1 -> BC/7  "testSig_CoEng_stOld"
  spec_CoEng_tiNormal/1 -> BC/8  "testSig_CoEng_tiNormal"
  spec_CoEng_tiStandby/1 -> BC/9  "testSig_CoEng_tiStandby"
  spec_CoEng_tiStart/1 -> BC/10  "testSig_CoEng_tiStart"
  spec_CoEng_tiAfterrun/1 -> BC/11  "testSig_CoEng_tiAfterrun"
  spec_CoEng_tiNrml2Strt_mp/1 -> BC/12  "testSig_CoEng_tiNrml2Strt_mp"

== system TST_CoEng_StEng/simulationInput/testSignals_R004 ==
  BC : BusCreator  Inputs=12
  spec_CoEng_st : FromWorkspace  VariableName=testSig_CoEng_st  Interpolate=off  OutputAfterFinalValue=Holding final value
  spec_CoEng_stOld : FromWorkspace  VariableName=testSig_CoEng_stOld  Interpolate=off  OutputAfterFinalValue=Holding final value
  spec_CoEng_tiAfterrun : FromWorkspace  VariableName=testSig_CoEng_tiAfterrun  Interpolate=off  OutputAfterFinalValue=Holding final value
  spec_CoEng_tiNormal : FromWorkspace  VariableName=testSig_CoEng_tiNormal  Interpolate=off  OutputAfterFinalValue=Holding final value
  spec_CoEng_tiNrml2Strt_mp : FromWorkspace  VariableName=testSig_CoEng_tiNrml2Strt_mp  Interpolate=off  OutputAfterFinalValue=Holding final value
  spec_CoEng_tiStandby : FromWorkspace  VariableName=testSig_CoEng_tiStandby  Interpolate=off  OutputAfterFinalValue=Holding final value
  spec_CoEng_tiStart : FromWorkspace  VariableName=testSig_CoEng_tiStart  Interpolate=off  OutputAfterFinalValue=Holding final value
  spec_DSM_bCoEngNrml2Strt : FromWorkspace  VariableName=testSig_DSM_bCoEngNrml2Strt  Interpolate=off  OutputAfterFinalValue=Holding final value
  spec_Epm_nEng : FromWorkspace  VariableName=testSig_Epm_nEng  Interpolate=off  OutputAfterFinalValue=Holding final value
  spec_StSys_stStrt : FromWorkspace  VariableName=testSig_StSys_stStrt  Interpolate=off  OutputAfterFinalValue=Holding final value
  spec_SyC_stPostDrv : FromWorkspace  VariableName=testSig_SyC_stPostDrv  Interpolate=off  OutputAfterFinalValue=Holding final value
  spec_T15_st : FromWorkspace  VariableName=testSig_T15_st  Interpolate=off  OutputAfterFinalValue=Holding final value
  testSignals : Outport
  wires:
  BC/1 -> testSignals/1
  spec_T15_st/1 -> BC/1  "testSig_T15_st"
  spec_Epm_nEng/1 -> BC/2  "testSig_Epm_nEng"
  spec_StSys_stStrt/1 -> BC/3  "testSig_StSys_stStrt"
  spec_SyC_stPostDrv/1 -> BC/4  "testSig_SyC_stPostDrv"
  spec_DSM_bCoEngNrml2Strt/1 -> BC/5  "testSig_DSM_bCoEngNrml2Strt"
  spec_CoEng_st/1 -> BC/6  "testSig_CoEng_st"
  spec_CoEng_stOld/1 -> BC/7  "testSig_CoEng_stOld"
  spec_CoEng_tiNormal/1 -> BC/8  "testSig_CoEng_tiNormal"
  spec_CoEng_tiStandby/1 -> BC/9  "testSig_CoEng_tiStandby"
  spec_CoEng_tiStart/1 -> BC/10  "testSig_CoEng_tiStart"
  spec_CoEng_tiAfterrun/1 -> BC/11  "testSig_CoEng_tiAfterrun"
  spec_CoEng_tiNrml2Strt_mp/1 -> BC/12  "testSig_CoEng_tiNrml2Strt_mp"

== system TST_CoEng_StEng/simulationInput/testSignals_R005 ==
  BC : BusCreator  Inputs=12
  spec_CoEng_st : FromWorkspace  VariableName=testSig_CoEng_st  Interpolate=off  OutputAfterFinalValue=Holding final value
  spec_CoEng_stOld : FromWorkspace  VariableName=testSig_CoEng_stOld  Interpolate=off  OutputAfterFinalValue=Holding final value
  spec_CoEng_tiAfterrun : FromWorkspace  VariableName=testSig_CoEng_tiAfterrun  Interpolate=off  OutputAfterFinalValue=Holding final value
  spec_CoEng_tiNormal : FromWorkspace  VariableName=testSig_CoEng_tiNormal  Interpolate=off  OutputAfterFinalValue=Holding final value
  spec_CoEng_tiNrml2Strt_mp : FromWorkspace  VariableName=testSig_CoEng_tiNrml2Strt_mp  Interpolate=off  OutputAfterFinalValue=Holding final value
  spec_CoEng_tiStandby : FromWorkspace  VariableName=testSig_CoEng_tiStandby  Interpolate=off  OutputAfterFinalValue=Holding final value
  spec_CoEng_tiStart : FromWorkspace  VariableName=testSig_CoEng_tiStart  Interpolate=off  OutputAfterFinalValue=Holding final value
  spec_DSM_bCoEngNrml2Strt : FromWorkspace  VariableName=testSig_DSM_bCoEngNrml2Strt  Interpolate=off  OutputAfterFinalValue=Holding final value
  spec_Epm_nEng : FromWorkspace  VariableName=testSig_Epm_nEng  Interpolate=off  OutputAfterFinalValue=Holding final value
  spec_StSys_stStrt : FromWorkspace  VariableName=testSig_StSys_stStrt  Interpolate=off  OutputAfterFinalValue=Holding final value
  spec_SyC_stPostDrv : FromWorkspace  VariableName=testSig_SyC_stPostDrv  Interpolate=off  OutputAfterFinalValue=Holding final value
  spec_T15_st : FromWorkspace  VariableName=testSig_T15_st  Interpolate=off  OutputAfterFinalValue=Holding final value
  testSignals : Outport
  wires:
  BC/1 -> testSignals/1
  spec_T15_st/1 -> BC/1  "testSig_T15_st"
  spec_Epm_nEng/1 -> BC/2  "testSig_Epm_nEng"
  spec_StSys_stStrt/1 -> BC/3  "testSig_StSys_stStrt"
  spec_SyC_stPostDrv/1 -> BC/4  "testSig_SyC_stPostDrv"
  spec_DSM_bCoEngNrml2Strt/1 -> BC/5  "testSig_DSM_bCoEngNrml2Strt"
  spec_CoEng_st/1 -> BC/6  "testSig_CoEng_st"
  spec_CoEng_stOld/1 -> BC/7  "testSig_CoEng_stOld"
  spec_CoEng_tiNormal/1 -> BC/8  "testSig_CoEng_tiNormal"
  spec_CoEng_tiStandby/1 -> BC/9  "testSig_CoEng_tiStandby"
  spec_CoEng_tiStart/1 -> BC/10  "testSig_CoEng_tiStart"
  spec_CoEng_tiAfterrun/1 -> BC/11  "testSig_CoEng_tiAfterrun"
  spec_CoEng_tiNrml2Strt_mp/1 -> BC/12  "testSig_CoEng_tiNrml2Strt_mp"

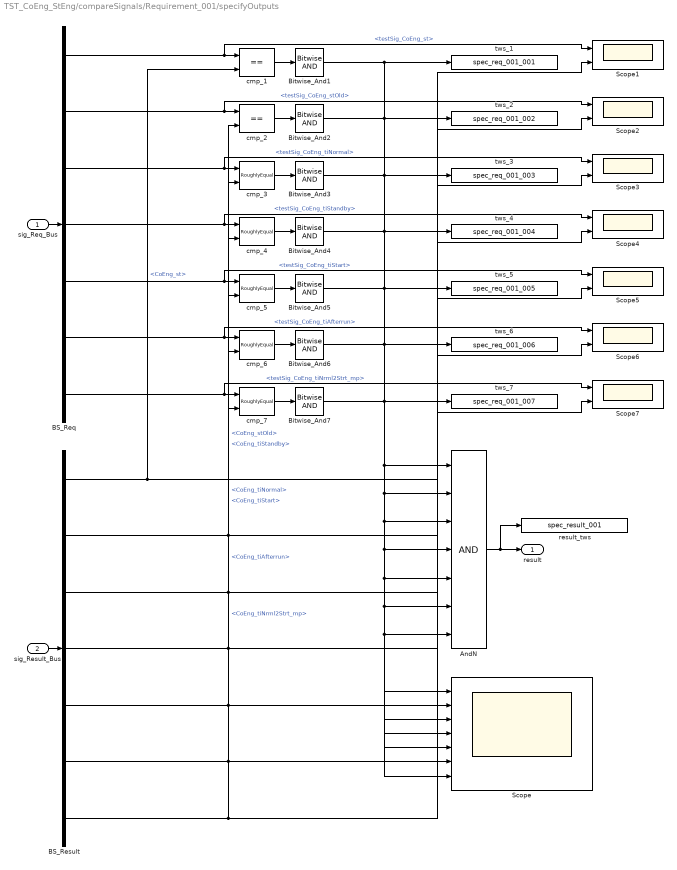
== system TST_CoEng_StEng/compareSignals/Requirement_001/specifyOutputs ==
  sig_Req_Bus : Inport
  sig_Result_Bus : Inport  Port=2
  AndN : Logic  Inputs=7
  BS_Req : BusSelector  OutputSignals=testSig_CoEng_st,testSig_CoEng_stOld,testSig_CoEng_tiNormal,testSig_CoEng_tiStandby,testSig_CoEng_tiStart,testSig_CoEng_tiAfterrun,testSig_CoEng_tiNrml2Strt_mp
  BS_Result : BusSelector  OutputSignals=CoEng_st,CoEng_stOld,CoEng_tiNormal,CoEng_tiStandby,CoEng_tiStart,CoEng_tiAfterrun,CoEng_tiNrml2Strt_mp
  Bitwise_And{1..7} (7 alike) : simulink/Logic and Bit Operations/Bitwise Operator  logicop=AND  UseBitMask=off  BitMask=bin2dec('11011001')  BitMaskRealWorld=Stored Integer
  Scope : Scope  NumInputPorts=7
  Scope{1..7} (7 alike) : Scope  NumInputPorts=2
  cmp_1 : RelationalOperator  Operator===  RndMeth=Nearest  InputSameDT=on
  cmp_2 : RelationalOperator  Operator===  RndMeth=Nearest  InputSameDT=on
  cmp_{3..7} (5 alike) : UnitTest_Lib/RoughlyEqual  slope=0.1
  result_tws : ToWorkspace  VariableName=spec_result_001
  tws_1 : ToWorkspace  VariableName=spec_req_001_001
  tws_2 : ToWorkspace  VariableName=spec_req_001_002
  tws_3 : ToWorkspace  VariableName=spec_req_001_003
  tws_4 : ToWorkspace  VariableName=spec_req_001_004
  tws_5 : ToWorkspace  VariableName=spec_req_001_005
  tws_6 : ToWorkspace  VariableName=spec_req_001_006
  tws_7 : ToWorkspace  VariableName=spec_req_001_007
  result : Outport
  wires:
  sig_Req_Bus/1 -> BS_Req/1
  sig_Result_Bus/1 -> BS_Result/1
  AndN/1 -> result/1, result_tws/1
  BS_Req/1 -> cmp_1/1, Scope1/1  "<testSig_CoEng_st>"
  BS_Result/1 -> cmp_1/2, Scope1/2  "<CoEng_st>"
  cmp_1/1 -> Bitwise_And1/1
  Bitwise_And1/1 -> AndN/1, Scope/1, tws_1/1
  BS_Req/2 -> cmp_2/1, Scope2/1  "<testSig_CoEng_stOld>"
  BS_Result/2 -> cmp_2/2, Scope2/2  "<CoEng_stOld>"
  cmp_2/1 -> Bitwise_And2/1
  Bitwise_And2/1 -> AndN/2, Scope/2, tws_2/1
  BS_Req/3 -> cmp_3/1, Scope3/1  "<testSig_CoEng_tiNormal>"
  BS_Result/3 -> cmp_3/2, Scope3/2  "<CoEng_tiNormal>"
  cmp_3/1 -> Bitwise_And3/1
  Bitwise_And3/1 -> AndN/3, Scope/3, tws_3/1
  BS_Req/4 -> cmp_4/1, Scope4/1  "<testSig_CoEng_tiStandby>"
  BS_Result/4 -> cmp_4/2, Scope4/2  "<CoEng_tiStandby>"
  cmp_4/1 -> Bitwise_And4/1
  Bitwise_And4/1 -> AndN/4, Scope/4, tws_4/1
  BS_Req/5 -> cmp_5/1, Scope5/1  "<testSig_CoEng_tiStart>"
  BS_Result/5 -> cmp_5/2, Scope5/2  "<CoEng_tiStart>"
  cmp_5/1 -> Bitwise_And5/1
  Bitwise_And5/1 -> AndN/5, Scope/5, tws_5/1
  BS_Req/6 -> cmp_6/1, Scope6/1  "<testSig_CoEng_tiAfterrun>"
  BS_Result/6 -> cmp_6/2, Scope6/2  "<CoEng_tiAfterrun>"
  cmp_6/1 -> Bitwise_And6/1
  Bitwise_And6/1 -> AndN/6, Scope/6, tws_6/1
  BS_Req/7 -> cmp_7/1, Scope7/1  "<testSig_CoEng_tiNrml2Strt_mp>"
  BS_Result/7 -> cmp_7/2, Scope7/2  "<CoEng_tiNrml2Strt_mp>"
  cmp_7/1 -> Bitwise_And7/1
  Bitwise_And7/1 -> AndN/7, Scope/7, tws_7/1

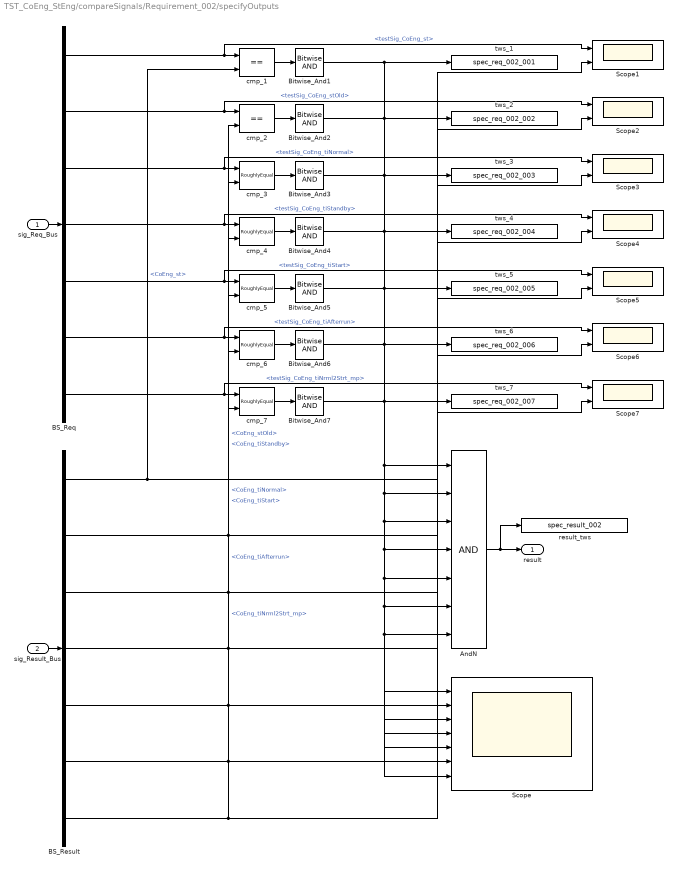
== system TST_CoEng_StEng/compareSignals/Requirement_002/specifyOutputs ==
  sig_Req_Bus : Inport
  sig_Result_Bus : Inport  Port=2
  AndN : Logic  Inputs=7
  BS_Req : BusSelector  OutputSignals=testSig_CoEng_st,testSig_CoEng_stOld,testSig_CoEng_tiNormal,testSig_CoEng_tiStandby,testSig_CoEng_tiStart,testSig_CoEng_tiAfterrun,testSig_CoEng_tiNrml2Strt_mp
  BS_Result : BusSelector  OutputSignals=CoEng_st,CoEng_stOld,CoEng_tiNormal,CoEng_tiStandby,CoEng_tiStart,CoEng_tiAfterrun,CoEng_tiNrml2Strt_mp
  Bitwise_And{1..7} (7 alike) : simulink/Logic and Bit Operations/Bitwise Operator  logicop=AND  UseBitMask=off  BitMask=bin2dec('11011001')  BitMaskRealWorld=Stored Integer
  Scope : Scope  NumInputPorts=7
  Scope{1..7} (7 alike) : Scope  NumInputPorts=2
  cmp_1 : RelationalOperator  Operator===  RndMeth=Nearest  InputSameDT=on
  cmp_2 : RelationalOperator  Operator===  RndMeth=Nearest  InputSameDT=on
  cmp_{3..7} (5 alike) : UnitTest_Lib/RoughlyEqual  slope=0.1
  result_tws : ToWorkspace  VariableName=spec_result_002
  tws_1 : ToWorkspace  VariableName=spec_req_002_001
  tws_2 : ToWorkspace  VariableName=spec_req_002_002
  tws_3 : ToWorkspace  VariableName=spec_req_002_003
  tws_4 : ToWorkspace  VariableName=spec_req_002_004
  tws_5 : ToWorkspace  VariableName=spec_req_002_005
  tws_6 : ToWorkspace  VariableName=spec_req_002_006
  tws_7 : ToWorkspace  VariableName=spec_req_002_007
  result : Outport
  wires:
  sig_Req_Bus/1 -> BS_Req/1
  sig_Result_Bus/1 -> BS_Result/1
  AndN/1 -> result/1, result_tws/1
  BS_Req/1 -> cmp_1/1, Scope1/1  "<testSig_CoEng_st>"
  BS_Result/1 -> cmp_1/2, Scope1/2  "<CoEng_st>"
  cmp_1/1 -> Bitwise_And1/1
  Bitwise_And1/1 -> AndN/1, Scope/1, tws_1/1
  BS_Req/2 -> cmp_2/1, Scope2/1  "<testSig_CoEng_stOld>"
  BS_Result/2 -> cmp_2/2, Scope2/2  "<CoEng_stOld>"
  cmp_2/1 -> Bitwise_And2/1
  Bitwise_And2/1 -> AndN/2, Scope/2, tws_2/1
  BS_Req/3 -> cmp_3/1, Scope3/1  "<testSig_CoEng_tiNormal>"
  BS_Result/3 -> cmp_3/2, Scope3/2  "<CoEng_tiNormal>"
  cmp_3/1 -> Bitwise_And3/1
  Bitwise_And3/1 -> AndN/3, Scope/3, tws_3/1
  BS_Req/4 -> cmp_4/1, Scope4/1  "<testSig_CoEng_tiStandby>"
  BS_Result/4 -> cmp_4/2, Scope4/2  "<CoEng_tiStandby>"
  cmp_4/1 -> Bitwise_And4/1
  Bitwise_And4/1 -> AndN/4, Scope/4, tws_4/1
  BS_Req/5 -> cmp_5/1, Scope5/1  "<testSig_CoEng_tiStart>"
  BS_Result/5 -> cmp_5/2, Scope5/2  "<CoEng_tiStart>"
  cmp_5/1 -> Bitwise_And5/1
  Bitwise_And5/1 -> AndN/5, Scope/5, tws_5/1
  BS_Req/6 -> cmp_6/1, Scope6/1  "<testSig_CoEng_tiAfterrun>"
  BS_Result/6 -> cmp_6/2, Scope6/2  "<CoEng_tiAfterrun>"
  cmp_6/1 -> Bitwise_And6/1
  Bitwise_And6/1 -> AndN/6, Scope/6, tws_6/1
  BS_Req/7 -> cmp_7/1, Scope7/1  "<testSig_CoEng_tiNrml2Strt_mp>"
  BS_Result/7 -> cmp_7/2, Scope7/2  "<CoEng_tiNrml2Strt_mp>"
  cmp_7/1 -> Bitwise_And7/1
  Bitwise_And7/1 -> AndN/7, Scope/7, tws_7/1

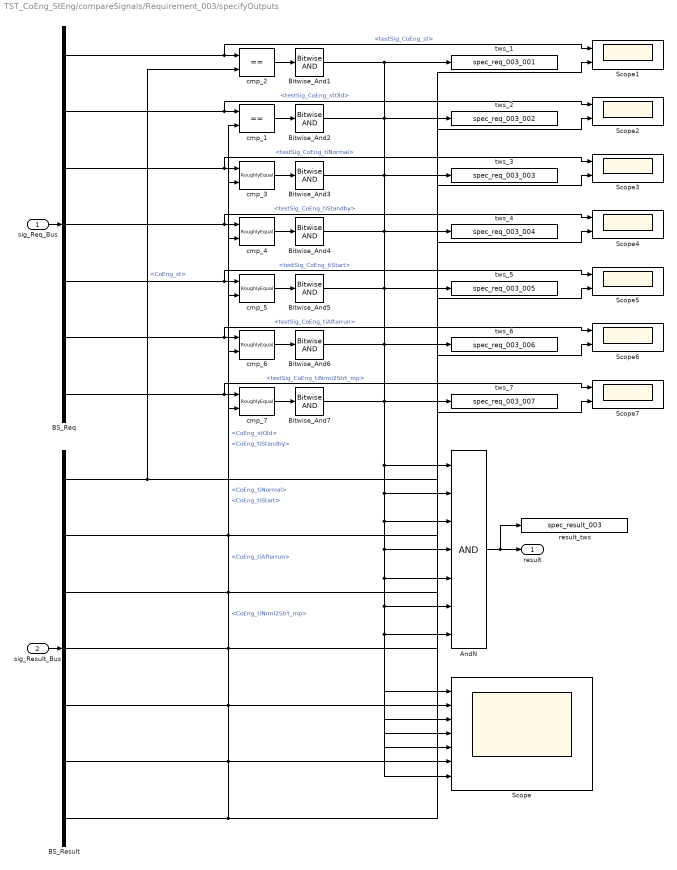
== system TST_CoEng_StEng/compareSignals/Requirement_003/specifyOutputs ==
  sig_Req_Bus : Inport
  sig_Result_Bus : Inport  Port=2
  AndN : Logic  Inputs=7
  BS_Req : BusSelector  OutputSignals=testSig_CoEng_st,testSig_CoEng_stOld,testSig_CoEng_tiNormal,testSig_CoEng_tiStandby,testSig_CoEng_tiStart,testSig_CoEng_tiAfterrun,testSig_CoEng_tiNrml2Strt_mp
  BS_Result : BusSelector  OutputSignals=CoEng_st,CoEng_stOld,CoEng_tiNormal,CoEng_tiStandby,CoEng_tiStart,CoEng_tiAfterrun,CoEng_tiNrml2Strt_mp
  Bitwise_And{1..7} (7 alike) : simulink/Logic and Bit Operations/Bitwise Operator  logicop=AND  UseBitMask=off  BitMask=bin2dec('11011001')  BitMaskRealWorld=Stored Integer
  Scope : Scope  NumInputPorts=7
  Scope{1..7} (7 alike) : Scope  NumInputPorts=2
  cmp_1 : RelationalOperator  Operator===  RndMeth=Nearest  InputSameDT=on
  cmp_2 : RelationalOperator  Operator===  RndMeth=Nearest  InputSameDT=on
  cmp_{3..7} (5 alike) : UnitTest_Lib/RoughlyEqual  slope=0.1
  result_tws : ToWorkspace  VariableName=spec_result_003
  tws_1 : ToWorkspace  VariableName=spec_req_003_001
  tws_2 : ToWorkspace  VariableName=spec_req_003_002
  tws_3 : ToWorkspace  VariableName=spec_req_003_003
  tws_4 : ToWorkspace  VariableName=spec_req_003_004
  tws_5 : ToWorkspace  VariableName=spec_req_003_005
  tws_6 : ToWorkspace  VariableName=spec_req_003_006
  tws_7 : ToWorkspace  VariableName=spec_req_003_007
  result : Outport
  wires:
  sig_Req_Bus/1 -> BS_Req/1
  sig_Result_Bus/1 -> BS_Result/1
  AndN/1 -> result/1, result_tws/1
  BS_Req/1 -> cmp_2/1, Scope1/1  "<testSig_CoEng_st>"
  BS_Result/1 -> cmp_2/2, Scope1/2  "<CoEng_st>"
  cmp_2/1 -> Bitwise_And1/1
  Bitwise_And1/1 -> AndN/1, Scope/1, tws_1/1
  BS_Req/2 -> cmp_1/1, Scope2/1  "<testSig_CoEng_stOld>"
  BS_Result/2 -> cmp_1/2, Scope2/2  "<CoEng_stOld>"
  cmp_1/1 -> Bitwise_And2/1
  Bitwise_And2/1 -> AndN/2, Scope/2, tws_2/1
  BS_Req/3 -> cmp_3/1, Scope3/1  "<testSig_CoEng_tiNormal>"
  BS_Result/3 -> cmp_3/2, Scope3/2  "<CoEng_tiNormal>"
  cmp_3/1 -> Bitwise_And3/1
  Bitwise_And3/1 -> AndN/3, Scope/3, tws_3/1
  BS_Req/4 -> cmp_4/1, Scope4/1  "<testSig_CoEng_tiStandby>"
  BS_Result/4 -> cmp_4/2, Scope4/2  "<CoEng_tiStandby>"
  cmp_4/1 -> Bitwise_And4/1
  Bitwise_And4/1 -> AndN/4, Scope/4, tws_4/1
  BS_Req/5 -> cmp_5/1, Scope5/1  "<testSig_CoEng_tiStart>"
  BS_Result/5 -> cmp_5/2, Scope5/2  "<CoEng_tiStart>"
  cmp_5/1 -> Bitwise_And5/1
  Bitwise_And5/1 -> AndN/5, Scope/5, tws_5/1
  BS_Req/6 -> cmp_6/1, Scope6/1  "<testSig_CoEng_tiAfterrun>"
  BS_Result/6 -> cmp_6/2, Scope6/2  "<CoEng_tiAfterrun>"
  cmp_6/1 -> Bitwise_And6/1
  Bitwise_And6/1 -> AndN/6, Scope/6, tws_6/1
  BS_Req/7 -> cmp_7/1, Scope7/1  "<testSig_CoEng_tiNrml2Strt_mp>"
  BS_Result/7 -> cmp_7/2, Scope7/2  "<CoEng_tiNrml2Strt_mp>"
  cmp_7/1 -> Bitwise_And7/1
  Bitwise_And7/1 -> AndN/7, Scope/7, tws_7/1
